simulink library "doLib"  (R2018a)
settings: Solver=VariableStepAuto  StartTime=0.0  StopTime=10.0  RelTol=1e-3  EnableMultiTasking=on
undefined symbols (not defined in the file): DiscIntNeverNeededParam, NumBits1, NumBits2, SlciDemosColors, Slope1, Slope2
libraries: simulink x26, simulink_need_slupdate x12, slcilib x1
settings Model: Creator=rsnah  LastModifiedBy=bpotter
settings DataIOCC: LimitDataPoints=on
settings OptimizationCC: LifeSpan=inf
settings DebuggingCC: AllowSymbolicDim=off  SFUnexpectedBacktrackingDiag=warning  SFNoUnconditionalDefaultTransitionDiag=warning  SFExecutionAtInitializationDiag=none
settings ModelReferenceCC: PropagateSignalLabelsOutOfModel=off
settings CodeAppCC: StateflowObjectComments=on
settings GRTTargetCC: TargetLangStandard=C89/C90 (ANSI)
settings ConfigComp: CovMetricSettings=dw  CovHtmlReporting=on  CovSaveCumulativeToWorkspaceVar=on  CovSaveSingleToWorkspaceVar=on  CovExternalEMLEnable=off

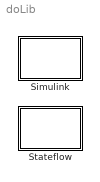
== system doLib ==
  Simulink : Subsystem
  Stateflow : Subsystem

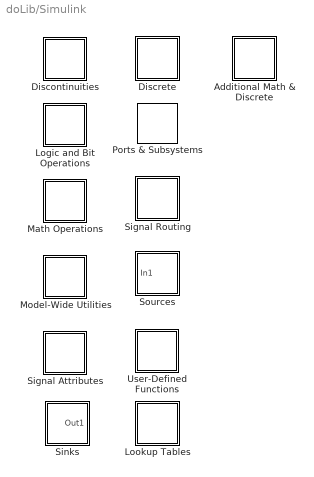
== system doLib/Simulink ==
  Additional Math & Discrete : Subsystem
      mask Display: image('additional_math_discrete.bmp')
  Discontinuities : Subsystem
      mask Display: image('nonlinear.bmp')
  Discrete : Subsystem
      mask Display: image('discrete.bmp')
  Logic and Bit Operations : Subsystem
      mask Display: image('logical_bit.bmp')
  Lookup Tables : Subsystem
      mask Display: image('tables.bmp')
  Math Operations : Subsystem
      mask Display: image('math.bmp')
  Model-Wide Utilities : Subsystem
      mask Display:
      | image('blank_block.bmp')
      | color('darkBlue')
      | disp('Misc')
  Ports & Subsystems : slcilib/Simulink/Ports & Subsystems  SystemSampleTime=-1
      settings: SourceProductName=Simulink Code Inspector  SourceProductBaseCode=CI
  Signal Attributes : Subsystem
      mask Display: image('attributes.bmp')
  Signal Routing : Subsystem
      mask Display: image('signals.bmp')
  Sinks : Subsystem
      mask Display: image('sinks.bmp')
  Sources : Subsystem
      mask Display: image('sources.bmp')
  User-Defined Functions : Subsystem
      mask Display: image('functions.bmp')

== system doLib/Stateflow ==
  Chart : Stateflow chart  TreatAsAtomicUnit=on
      settings: RTWSystemCode=Inline

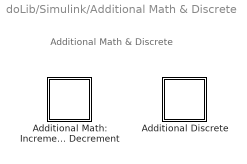
== system doLib/Simulink/Additional Math & Discrete ==
  note: Additional Math & Discrete
  Additional Discrete : Subsystem
      mask Display: image('discrete.bmp')
  Additional Math: Increment - Decrement : Subsystem
      mask Display: image('increment_decrement.bmp')

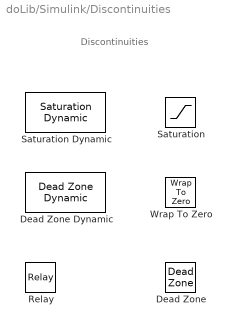
== system doLib/Simulink/Discontinuities ==
  note: Discontinuities
  Dead Zone : DeadZone
  Dead Zone Dynamic : simulink/Discontinuities/Dead Zone Dynamic
      settings: SourceProductName=Simulink  SourceProductBaseCode=SL
  Relay : Relay
  Saturation : Saturate
  Saturation Dynamic : simulink/Discontinuities/Saturation Dynamic  OutMin=[]  OutMax=[]  OutDataTypeStr=Inherit: Same as second input  OutDataType=fixdt(1, 16)  OutScaling=2^-10  DoSatur=off
  Wrap To Zero : simulink/Discontinuities/Wrap To Zero  Threshold=255
      settings: SourceProductName=Simulink  SourceProductBaseCode=SL

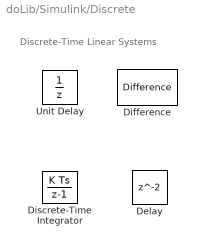
== system doLib/Simulink/Discrete ==
  note: Discrete-Time Linear Systems
  Delay : Delay
  Difference : simulink/Discrete/Difference  ICPrevInput=0.0  InputProcessing=Inherited  OutMin=[]  OutMax=[]  OutDataType=fixdt(1, 16)  OutScaling=2^-10  DoSatur=off
  Discrete-Time Integrator : DiscreteIntegrator  SampleTime=-1  ICPrevOutput=DiscIntNeverNeededParam  ICPrevScaledInput=DiscIntNeverNeededParam
  Unit Delay : UnitDelay  SampleTime=-1

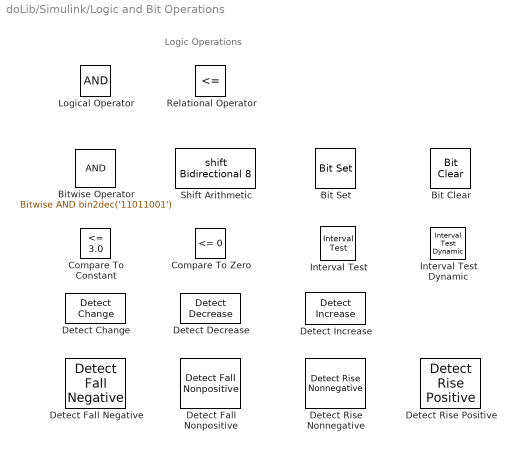
== system doLib/Simulink/Logic and Bit Operations ==
  note: Logic Operations
  Bit Clear : simulink/Logic and Bit Operations/Bit Clear  iBit=0
      settings: SourceProductName=Simulink  SourceProductBaseCode=SL
  Bit Set : simulink/Logic and Bit Operations/Bit Set  iBit=0
      settings: SourceProductName=Simulink  SourceProductBaseCode=SL
  Bitwise Operator : simulink/Logic and Bit Operations/Bitwise Operator  logicop=AND  UseBitMask=on  BitMask=bin2dec('11011001')  BitMaskRealWorld=Stored Integer
  Compare To Constant : simulink/Logic and Bit Operations/Compare To Constant  relop=<=  const=3.0  OutDataTypeStr=boolean
  Compare To Zero : simulink/Logic and Bit Operations/Compare To Zero  relop=<=  OutDataTypeStr=boolean
  Detect Change : simulink/Logic and Bit Operations/Detect Change  vinit=0  InputProcessing=Inherited  OutDataTypeStr=boolean
  Detect Decrease : simulink/Logic and Bit Operations/Detect Decrease  vinit=0.0  InputProcessing=Inherited  OutDataTypeStr=boolean
  Detect Fall Negative : simulink/Logic and Bit Operations/Detect Fall Negative  vinit=0  InputProcessing=Inherited  OutDataTypeStr=boolean
      settings: SourceProductName=Simulink  SourceProductBaseCode=SL
  Detect Fall Nonpositive : simulink/Logic and Bit Operations/Detect Fall Nonpositive  vinit=0  InputProcessing=Inherited  OutDataTypeStr=boolean
      settings: SourceProductName=Simulink  SourceProductBaseCode=SL
  Detect Increase : simulink/Logic and Bit Operations/Detect Increase  vinit=0.0  InputProcessing=Inherited  OutDataTypeStr=boolean
  Detect Rise Nonnegative : simulink/Logic and Bit Operations/Detect Rise Nonnegative  vinit=0  InputProcessing=Inherited  OutDataTypeStr=boolean
      settings: SourceProductName=Simulink  SourceProductBaseCode=SL
  Detect Rise Positive : simulink/Logic and Bit Operations/Detect Rise Positive  vinit=0  InputProcessing=Inherited  OutDataTypeStr=boolean
  Interval Test : simulink/Logic and Bit Operations/Interval Test  IntervalClosedRight=on  uplimit=0.5  IntervalClosedLeft=on  lowlimit=-0.5  OutDataTypeStr=boolean
  Interval Test Dynamic : simulink/Logic and Bit Operations/Interval Test Dynamic  IntervalClosedRight=on  IntervalClosedLeft=on  OutDataTypeStr=boolean
      settings: SourceProductName=Simulink  SourceProductBaseCode=SL
  Logical Operator : Logic  AllPortsSameDT=off  OutDataTypeStr=boolean
  Relational Operator : RelationalOperator  Operator=<=  OutDataTypeStr=boolean  RndMeth=Nearest  InputSameDT=on
  Shift Arithmetic : ArithShift  BitShiftNumber=8  DiagnosticForOORShift=Error
      settings: CopyFcn=set_param(gcb,'LinkStatus','none'); set_param(gcb,'Mask','off'); set_param(gcb,'MaskType',''); set_param(gcb,'MaskDescription',''); set_param(gcb,'OpenFcn',''); set_param(gcb,'CopyFcn','')

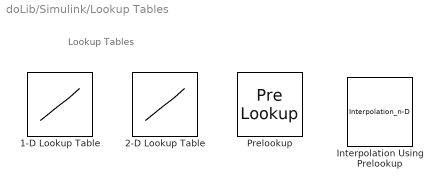
== system doLib/Simulink/Lookup Tables ==
  note: Lookup Tables
  1-D Lookup Table : Lookup_n-D  NumberOfTableDimensions=1  LookupTableObject=''  BreakpointsForDimension1=[-3 -2 -1 0 1 2 3]  Table=[-5 -4 -1 0 1 4 5]  ExtrapMethod=Clip  RemoveProtectionInput=on  UseLastTableValue=on  RndMeth=Zero  FractionDataTypeStr=double  InputSameDT=on
  2-D Lookup Table : Lookup_n-D  LookupTableObject=''  BreakpointsForDimension1=[1 2 3]  BreakpointsForDimension2=[1 2 3]  ExtrapMethod=Clip  RemoveProtectionInput=on  UseLastTableValue=on  RndMeth=Zero  FractionDataTypeStr=double  InputSameDT=on
  Interpolation Using Prelookup : Interpolation_n-D
  Prelookup : PreLookup  BreakpointsData=[10:10:110]  ExtrapMethod=Linear

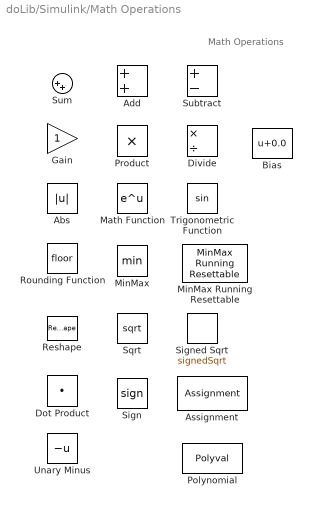
== system doLib/Simulink/Math Operations ==
  note: Math Operations
  Abs : Abs
  Add : Sum  InputSameDT=on  OutDataTypeStr=Inherit: Same as first input
  Assignment : Assignment  IndexOptions=Index vector (port)  Indices=1  OutputSizes=1
  Bias : Bias  Bias=0.0
  Divide : Product  Inputs=*/  OutDataTypeStr=Inherit: Same as first input
  Dot Product : DotProduct  InputSameDT=on  OutDataTypeStr=Inherit: Inherit via internal rule
  Gain : Gain  OutDataTypeStr=Inherit: Same as input  ParamDataTypeStr=Inherit: Same as input
  Math Function : Math  SaturateOnIntegerOverflow=on
  MinMax : MinMax  Inputs=2  InputSameDT=on
  MinMax Running Resettable : simulink/Math Operations/MinMax Running Resettable  Function=min  vinit=0.0
  Polynomial : Polyval  Coefs=[ +2.081618890e-019, -1.441693666e-014, +4.719686976e-010, -8.536869453e-006, +1.621573104e-001, -8.087801117e+001 ]
  Product : Product  RndMeth=Zero  InputSameDT=on  OutDataTypeStr=Inherit: Same as first input
  Reshape : Reshape
  Rounding Function : Rounding
  Sign : Signum
  Signed Sqrt : Sqrt  Operator=signedSqrt  SaturateOnIntegerOverflow=on
  Sqrt : Sqrt  SaturateOnIntegerOverflow=on
  Subtract : Sum  Inputs=+-  InputSameDT=on  OutDataTypeStr=Inherit: Same as first input
  Sum : Sum  Inputs=|++  InputSameDT=on  OutDataTypeStr=Inherit: Same as first input
  Trigonometric Function : Trigonometry
  Unary Minus : UnaryMinus

== system doLib/Simulink/Model-Wide Utilities ==
  note: Documentation
  DocBlock : simulink/Model-Wide Utilities/DocBlock  DocumentType=Text
  Model Info : simulink/Model-Wide Utilities/Model Info  Frame=on  DisplayStringWithTags=Model Info  HorizontalTextAlignment=Center  LeftAlignmentValue=0.5

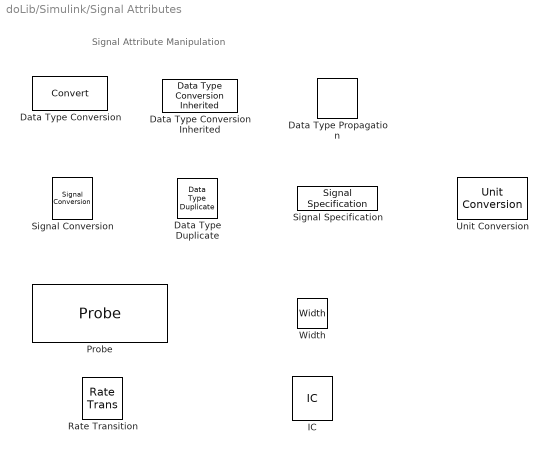
== system doLib/Simulink/Signal Attributes ==
  note: Signal Attribute Manipulation
  Data Type Duplicate : DataTypeDuplicate
  Data Type Conversion : DataTypeConversion
  Data Type Conversion Inherited : simulink/Signal Attributes/Data Type Conversion Inherited  ConvertRealWorld=Real World Value  DoSatur=off
      settings: SourceProductName=Simulink  SourceProductBaseCode=SL
  Data Type Propagation : simulink/Signal Attributes/Data Type Propagation  PropDataType=fixdt(1, 16)  IfRefDouble=double  IfRefSingle=single  IsSigned=IsSigned1 or IsSigned2  NumBitsBase=max([NumBits1 NumBits2])  NumBitsMult=1  NumBitsAdd=0  NumBitsAllowFinal=1:128  PropScaling=2^-10  ValuesUsedBestPrec=[5 -7]  SlopeBase=min([Slope1 Slope2])  SlopeMult=1  SlopeAdd=0  BiasBase=Bias1  BiasMult=1  BiasAdd=0
      settings: SourceProductName=Simulink  SourceProductBaseCode=SL
  IC : InitialCondition
  Probe : Probe  ProbeSignalDimensions=on  ProbeFramedSignal=on
  Rate Transition : RateTransition
  Signal Conversion : SignalConversion  OverrideOpt=on
  Signal Specification : SignalSpecification
  Unit Conversion : UnitConversion
  Width : Width

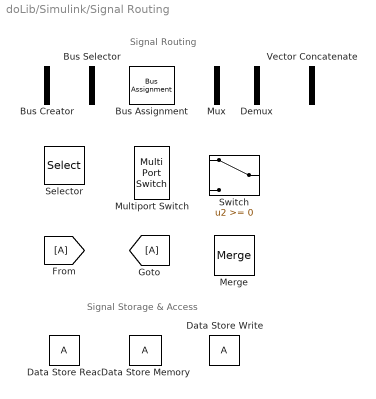
== system doLib/Simulink/Signal Routing ==
  note: Signal Routing
  note: Signal Storage & Access
  Bus Assignment : BusAssignment  AssignedSignals=signal1
  Bus Creator : BusCreator  Inputs=2
  Bus Selector : BusSelector  OutputSignals=signal1,signal2
  Data Store Memory : DataStoreMemory  ReadBeforeWriteMsg=warning  WriteAfterWriteMsg=warning  WriteAfterReadMsg=warning  ShowAdditionalParam=off
  Data Store Read : DataStoreRead
  Data Store Write : DataStoreWrite
  Demux : Demux  Outputs=2
  Merge : Merge  InitialOutput=0
  Multiport Switch : MultiPortSwitch  InputSameDT=on
  Mux : Mux  Inputs=2
  Selector : Selector  InputPortWidth=3  IndexOptions=Index vector (dialog)  Indices=[1 3]  OutputSizes=1
  Switch : Switch  InputSameDT=on
  Vector Concatenate : Concatenate

== system doLib/Simulink/Sinks ==
  note: Model & Subsystem Outputs
  Terminator : Terminator
  Out1 : Outport

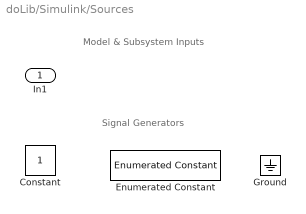
== system doLib/Simulink/Sources ==
  note: Model & Subsystem Inputs
  note: Signal Generators
  In1 : Inport
  Constant : Constant
  Enumerated Constant : simulink/Sources/Enumerated Constant  OutDataTypeStr=Enum: SlciDemosColors  Value=SlciDemosColors.Red  SampleTime=inf
      settings: SourceProductName=Simulink
  Ground : Ground

== system doLib/Simulink/User-Defined Functions ==
  note: User-defined Functions
  MATLAB Function : MATLAB Function  TreatAsAtomicUnit=on
      settings: RTWSystemCode=Inline
  More Info : Subsystem
      settings: OpenFcn=helpview([docroot '/mapfiles/simulink.map'],'legacy_code_tool','CSHelpWindow');
      mask Display: disp('Note: \n Simulink Code Inspector supports S-functions \n created by the Legacy Code Tool. ')

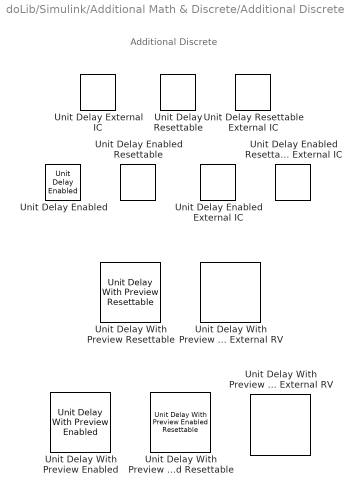
== system doLib/Simulink/Additional Math & Discrete/Additional Discrete ==
  note: Additional Discrete
  Unit Delay Enabled : simulink_need_slupdate/Unit Delay Enabled  vinit=0.0  tsamp=-1
      settings: SourceProductName=Simulink  SourceProductBaseCode=SL
  Unit Delay Enabled External IC : simulink_need_slupdate/Unit Delay Enabled External IC  tsamp=-1
      settings: SourceProductName=Simulink  SourceProductBaseCode=SL
  Unit Delay Enabled Resettable : simulink_need_slupdate/Unit Delay Enabled Resettable  vinit=0.0  tsamp=-1
      settings: SourceProductName=Simulink  SourceProductBaseCode=SL
  Unit Delay Enabled Resettable External IC : simulink_need_slupdate/Unit Delay Enabled Resettable External IC  tsamp=-1
      settings: SourceProductName=Simulink  SourceProductBaseCode=SL
  Unit Delay External IC : simulink_need_slupdate/Unit Delay External IC  tsamp=-1
      settings: SourceProductName=Simulink  SourceProductBaseCode=SL
  Unit Delay Resettable : simulink_need_slupdate/Unit Delay Resettable  vinit=0.0  tsamp=-1
      settings: SourceProductName=Simulink  SourceProductBaseCode=SL
  Unit Delay Resettable External IC : simulink_need_slupdate/Unit Delay Resettable External IC  tsamp=-1
      settings: SourceProductName=Simulink  SourceProductBaseCode=SL
  Unit Delay With Preview Enabled : simulink_need_slupdate/Unit Delay With Preview Enabled  vinit=0.0  tsamp=-1
      settings: SourceProductName=Simulink  SourceProductBaseCode=SL
  Unit Delay With Preview Enabled Resettable : simulink_need_slupdate/Unit Delay With Preview Enabled Resettable  vinit=0.0  tsamp=-1
      settings: SourceProductName=Simulink  SourceProductBaseCode=SL
  Unit Delay With Preview Enabled Resettable External RV : simulink_need_slupdate/Unit Delay With Preview Enabled Resettable External RV  vinit=0.0  tsamp=-1
      settings: SourceProductName=Simulink  SourceProductBaseCode=SL
  Unit Delay With Preview Resettable : simulink_need_slupdate/Unit Delay With Preview Resettable  vinit=0.0  tsamp=-1
      settings: SourceProductName=Simulink  SourceProductBaseCode=SL
  Unit Delay With Preview Resettable External RV : simulink_need_slupdate/Unit Delay With Preview Resettable External RV  vinit=0.0  tsamp=-1
      settings: SourceProductName=Simulink  SourceProductBaseCode=SL

== system doLib/Simulink/Additional Math & Discrete/Additional Math: Increment - Decrement ==
  note: Increment/Decrement
  Decrement Real World : simulink/Additional Math & Discrete/Additional Math: Increment - Decrement/Decrement Real World
      settings: SourceProductName=Simulink  SourceProductBaseCode=SL
  Increment Real World : simulink/Additional Math & Discrete/Additional Math: Increment - Decrement/Increment Real World
      settings: SourceProductName=Simulink  SourceProductBaseCode=SL

== system doLib/Simulink/User-Defined Functions/More Info ==

== stateflow chart doLib/Stateflow/Chart ==
  note: The Simulink Code Inspector supports the following subset of Stateflow:
      | \bullet Control flow constructed using the Stateflow Decision patterns
      | \bullet Data of all scope
      | \bullet Function-call output events
      | \bullet Hierarchically nested states
  (default) -> (junction 1) : /* Sign Function */
  (junction 1) -> (junction 4) [order 1] : [u < 0]
  (junction 1) -> (junction 3) [order 2]
  (junction 4) -> (junction 5) : {y = -1;}
  (junction 3) -> (junction 6) [order 1] : [u == 0]
  (junction 3) -> (junction 2) [order 2] : {y = 1;}
  (junction 6) -> (junction 7) : {y = 0;}
  (junction 7) -> (junction 2)
  (junction 5) -> (junction 7)
  (junction 2) -> (junction 8)
  data: u input int32; y output int32

== matlab function doLib/Simulink/User-Defined Functions/MATLAB Function ==
  data: u input; y output
function y = fcn(u)
%#codegen

y = u;
